simulink model "Modelling"  (R2020a)
settings: Solver=ode4  StartTime=0.0  StopTime=30  FixedStep=0.001  RelTol=1e-3
PreLoadFcn:
  | ControllerToProject.m
values from neighbouring files (symbols this model uses):
  b = 1    [ControllerToProject.m]    (also in Parameters.m)
  g = 9.81    [ControllerToProject.m]    (also in Parameters.m = 9.82)
  l = 0.36022    [ControllerToProject.m]    (also in Parameters.m = 0.35)
  mc = 0.9+0.1    (= 1)    [ControllerToProject.m]    (also in Parameters.m = 0.9)
  mp = 0.08887    [ControllerToProject.m]    (also in Parameters.m = 0.1)
undefined symbols (not defined in the file or in its folder): sigbuilder_block
libraries: simulink x2
settings Model: Creator=Emil  LastModifiedBy=Emil
settings DebuggingCC: ArithmeticOperatorsInVariantConditions=warning
settings SFSimCC: CustomCodeUndefinedFunction=UseInterfaceOnly

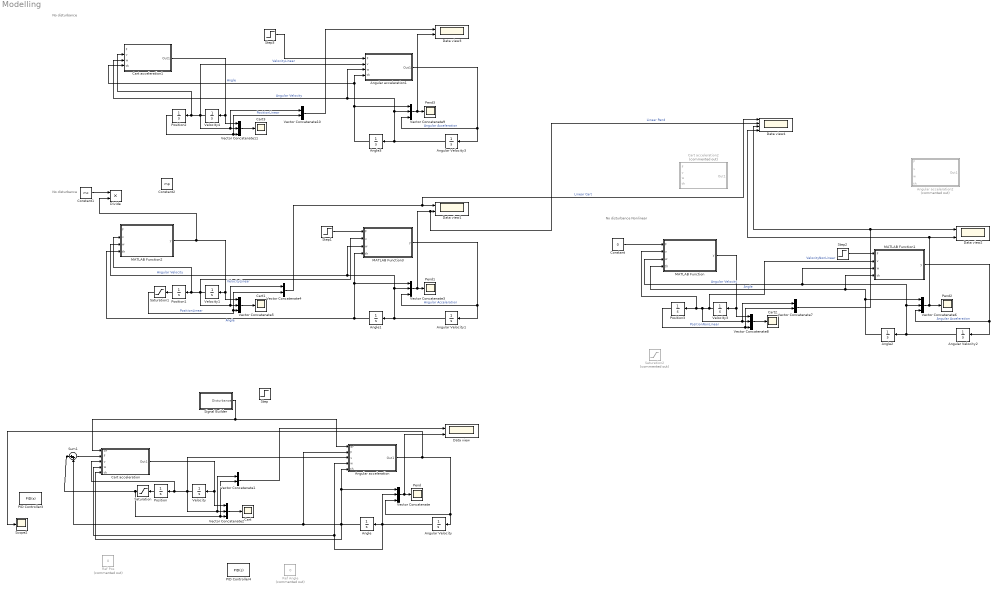
== system Modelling ==
  note: No disturbance
  note: No disturbance
      | Nonlinear
  note: No disturbance
  Angle{,1..3} (4 alike) : Integrator
  Angular Velocity{,1..3} (4 alike) : Integrator
  Angular acceleration : Subsystem
  Angular acceleration1 : Subsystem
  Angular acceleration2 : Subsystem  Commented=on
  Cart{,1..3} (4 alike) : Scope
  Cart acceleration : Subsystem
  Cart acceleration1 : Subsystem
  Cart acceleration2 : Subsystem  Commented=on
  Constant : Constant  Value=0
  Constant1 : Constant  Value=mc
  Constant2 : Constant  Value=mp
  Data view{,1..3} (4 alike) : Scope  NumInputPorts=2
  Data view4 : Scope  NumInputPorts=4
  Divide : Product  Inputs=**
  MATLAB Function : MATLAB Function  TreatAsAtomicUnit=on
  MATLAB Function1 : MATLAB Function  TreatAsAtomicUnit=on
  MATLAB Function2 : MATLAB Function  TreatAsAtomicUnit=on
  MATLAB Function3 : MATLAB Function  TreatAsAtomicUnit=on
  PID Controller3 : simulink/Continuous/PID Controller  Controller=PID  Form=Ideal  TimeDomain=Continuous-time  UseExternalTs=off  SampleTime=-1  IntegratorMethod=Forward Euler  FilterMethod=Forward Euler  ControllerParametersSource=internal  P=-380.892958771882  I=0.42148790930739  D=0.173217560929601  UseFilter=on  N=5979.02668424825  TunerSelectOption=Transfer Function Based (PID Tuner App)  InitialConditionSource=internal  InitialConditionForIntegrator=0  InitialConditionForFilter=0  DifferentiatorICPrevScaledInput=0  ExternalReset=none  TrackingMode=off  Kt=1  LimitOutput=on  UpperSaturationLimit=5  LowerSaturationLimit=-5  LinearizeAsGain=on  AntiWindupMode=clamping  Kb=1  POutMin=[]  POutMax=[]  IOutMin=[]  IOutMax=[]  DOutMin=[]  DOutMax=[]  NOutMin=[]  NOutMax=[]  SumOutMin=[]  SumOutMax=[]  SaturationOutMin=[]  SaturationOutMax=[]  PParamMin=[]  PParamMax=[]  IParamMin=[]  IParamMax=[]  DParamMin=[]  DParamMax=[]  NParamMin=[]  NParamMax=[]  KbParamMin=[]  KbParamMax=[]  KtParamMin=[]  KtParamMax=[]  KbOutMin=[]  KbOutMax=[]  KtOutMin=[]  KtOutMax=[]  IntegratorOutMin=[]  IntegratorOutMax=[]  FilterOutMin=[]  FilterOutMax=[]  SumI1OutMin=[]  SumI1OutMax=[]  SumI2OutMin=[]  SumI2OutMax=[]  SumI3OutMin=[]  SumI3OutMax=[]  SumI4OutMin=[]  SumI4OutMax=[]  SumDOutMin=[]  SumDOutMax=[]  DifferentiatorOutMin=[]  DifferentiatorOutMax=[]  FilterDiffOutCoefMin=[]  FilterDiffOutCoefMax=[]  ReciprocalOutMin=[]  ReciprocalOutMax=[]  SumDenOutMin=[]  SumDenOutMax=[]  SumNumOutMin=[]  SumNumOutMax=[]  DivideOutMin=[]  DivideOutMax=[]  UdiffTsProdOutMin=[]  UdiffTsProdOutMax=[]  NTsProdOutMin=[]  NTsProdOutMax=[]  UintegralTsProdOutMin=[]  UintegralTsProdOutMax=[]  UngainTsProdOutMin=[]  UngainTsProdOutMax=[]  IntegratorContinuousStateAttributes=''  IntegratorStateMustResolveToSignalObject=off  IntegratorRTWStateStorageClass=Auto  FilterContinuousStateAttributes=''  FilterStateMustResolveToSignalObject=off  FilterRTWStateStorageClass=Auto  ParallelPVariant=Passthrough  IdealPVariant=InternalParameters  IVariant=InternalParameters  DVariant=InternalParameters  IntegratorVariant=Continuous  SatVariant=Enabled  AWVariant=ContClampingIdeal  PCopyVariant=InternalParamsIdeal  TRVariant=Disabled  FdbkBlocksVariant=Forward  IdealPFdbkVariant=Disabled  SatFdbkVariant=Disabled  DerivativeFilterVariant=ContFilter  NVariant=InternalParameters  NCopyVariant=Disabled  FilterICVariant=InternalICsFilter  IntegratorICVariant=InternalICs  ExternalResetVariant=Disabled  TRSumVariant=Passthrough  SumFdbkVariant=Disabled  SumVariant=Sum_PID  TsampFilterVariant=InternalTs  TsampNgainVariant=Passthrough  TsampIntegralVariant=Passthrough
  PID Controller4 : simulink/Continuous/PID Controller  Controller=PID  Form=Ideal  TimeDomain=Continuous-time  UseExternalTs=off  SampleTime=-1  IntegratorMethod=Forward Euler  FilterMethod=Forward Euler  ControllerParametersSource=internal  P=-1.40813056601747  I=7297.16708467672  D=0  UseFilter=on  N=100  TunerSelectOption=Transfer Function Based (PID Tuner App)  InitialConditionSource=internal  InitialConditionForIntegrator=0  InitialConditionForFilter=0  DifferentiatorICPrevScaledInput=0  ExternalReset=none  TrackingMode=off  Kt=1  LimitOutput=on  UpperSaturationLimit=5  LowerSaturationLimit=-5  LinearizeAsGain=on  AntiWindupMode=clamping  Kb=1  POutMin=[]  POutMax=[]  IOutMin=[]  IOutMax=[]  DOutMin=[]  DOutMax=[]  NOutMin=[]  NOutMax=[]  SumOutMin=[]  SumOutMax=[]  SaturationOutMin=[]  SaturationOutMax=[]  PParamMin=[]  PParamMax=[]  IParamMin=[]  IParamMax=[]  DParamMin=[]  DParamMax=[]  NParamMin=[]  NParamMax=[]  KbParamMin=[]  KbParamMax=[]  KtParamMin=[]  KtParamMax=[]  KbOutMin=[]  KbOutMax=[]  KtOutMin=[]  KtOutMax=[]  IntegratorOutMin=[]  IntegratorOutMax=[]  FilterOutMin=[]  FilterOutMax=[]  SumI1OutMin=[]  SumI1OutMax=[]  SumI2OutMin=[]  SumI2OutMax=[]  SumI3OutMin=[]  SumI3OutMax=[]  SumI4OutMin=[]  SumI4OutMax=[]  SumDOutMin=[]  SumDOutMax=[]  DifferentiatorOutMin=[]  DifferentiatorOutMax=[]  FilterDiffOutCoefMin=[]  FilterDiffOutCoefMax=[]  ReciprocalOutMin=[]  ReciprocalOutMax=[]  SumDenOutMin=[]  SumDenOutMax=[]  SumNumOutMin=[]  SumNumOutMax=[]  DivideOutMin=[]  DivideOutMax=[]  UdiffTsProdOutMin=[]  UdiffTsProdOutMax=[]  NTsProdOutMin=[]  NTsProdOutMax=[]  UintegralTsProdOutMin=[]  UintegralTsProdOutMax=[]  UngainTsProdOutMin=[]  UngainTsProdOutMax=[]  IntegratorContinuousStateAttributes=''  IntegratorStateMustResolveToSignalObject=off  IntegratorRTWStateStorageClass=Auto  FilterContinuousStateAttributes=''  FilterStateMustResolveToSignalObject=off  FilterRTWStateStorageClass=Auto  ParallelPVariant=Passthrough  IdealPVariant=InternalParameters  IVariant=InternalParameters  DVariant=InternalParameters  IntegratorVariant=Continuous  SatVariant=Enabled  AWVariant=ContClampingIdeal  PCopyVariant=InternalParamsIdeal  TRVariant=Disabled  FdbkBlocksVariant=Forward  IdealPFdbkVariant=Disabled  SatFdbkVariant=Disabled  DerivativeFilterVariant=ContFilter  NVariant=InternalParameters  NCopyVariant=Disabled  FilterICVariant=InternalICsFilter  IntegratorICVariant=InternalICs  ExternalResetVariant=Disabled  TRSumVariant=Passthrough  SumFdbkVariant=Disabled  SumVariant=Sum_PID  TsampFilterVariant=InternalTs  TsampNgainVariant=Passthrough  TsampIntegralVariant=Passthrough
  Pend{,1..3} (4 alike) : Scope
  Position{,1..3} (4 alike) : Integrator
  Ref Angle : Constant  Commented=on  Value=0
  Ref Pos : Constant  Commented=on  Value=0
  Saturation : Saturate  UpperLimit=0.8  LowerLimit=-0.8  LinearizeAsGain=off
  Saturation1 : Saturate  UpperLimit=0.8  LowerLimit=-0.8
  Saturation2 : Saturate  Commented=on  UpperLimit=0.8  LowerLimit=-0.8
  Scope2 : Scope
  Signal Builder : Subsystem  Tag=STV Subsys  LoadFcn=sigbuilder_block('load');  StartFcn=sigbuilder_block('start');  StopFcn=sigbuilder_block('stop');  ClipboardFcn=sigbuilder_block('clipboard');  mask(Sigbuilder block){tuvar=[0:10]}
      mask help: Simulink:masks:SigbuilderBlock_MD
      mask init:
      | if ~strcmp(get_param(bdroot(gcbh),'SimulationStatus'),'stopped') tuvar = sigbuilder_block('maskInit'); end
      settings: CopyFcn=sigbuilder_block('copy');  DeleteFcn=sigbuilder_block('delete');  ModelCloseFcn=sigbuilder_block('modelClose');  PreSaveFcn=sigbuilder_block('preSave');  PauseFcn=sigbuilder_block('pause');  ContinueFcn=sigbuilder_block('continue');  NameChangeFcn=sigbuilder_block('namechange');  OpenFcn=sigbuilder_block('open',[6 30 1428 681.75 ]);  CloseFcn=sigbuilder_block('close');
      mask Display: plot(0, 0, 100, 100,[2, 2, 32, 32, 2], [68, 8, 8, 68, 68],[32, 2], [38, 38], [32, 19, 2],[53, 60, 44], [32, 17, 17, 2],[16, 16, 31, 31]);txt = getActiveGroup(gcbh);text(2, 100, txt,'verticalAlignment', 'top');
  Step : Step  Before=20  After=0  SampleTime=0
  Step1 : Step  Before=20  After=0  SampleTime=0
  Step2 : Step  Before=1  After=0  SampleTime=0
  Step3 : Step  Time=20  Before=1  After=0  SampleTime=0
  Sum1 : Sum  Inputs=|++
  Vector Concatenate{,2..3,5..6,8..9,11} (8 alike) : Concatenate  NumInputs=3
  Vector Concatenate{1,4,7,10} (4 alike) : Concatenate
  Velocity{,1,3..4} (4 alike) : Integrator
  wires:
  Position/1 -> Saturation/1
  Velocity/1 -> Angular acceleration/3(v), Vector Concatenate2/2, Vector Concatenate1/1, Position/1, Cart acceleration/3(v)
  Cart acceleration/1(Out1) -> Velocity/1, Vector Concatenate2/1
  Angular acceleration/1(Out1) -> Scope2/1, Vector Concatenate/3, Angular Velocity/1
  Angular Velocity/1 -> Vector Concatenate/2, Angle/1, Cart acceleration/4(w), Angular acceleration/4(w)
  Saturation/1 -> Sum1/1, Vector Concatenate1/2, Vector Concatenate2/3
  Angle/1 -> Angular acceleration/2(F), Sum1/2, Vector Concatenate/1, Angular acceleration/5(th), Cart acceleration/5(th)
  Vector Concatenate/1 -> Data view/2, Pend/1
  Vector Concatenate2/1 -> Cart/1
  Vector Concatenate1/1 -> Data view/1
  Signal Builder/1(Disturbance) -> Angular acceleration/1(dF), Cart acceleration/1(dF)
  Position1/1 -> Saturation1/1
  Vector Concatenate3/1 -> Data view4/2, Data view1/2, Pend1/1  "Linear Pend"
  Vector Concatenate4/1 -> Data view4/1, Data view1/1  "Linear Cart"
  Vector Concatenate5/1 -> Cart1/1
  Saturation1/1 -> Vector Concatenate4/2, Vector Concatenate5/3  "PositionLinear"
  Angular Velocity1/1 -> Vector Concatenate3/2, MATLAB Function3/3(w), MATLAB Function2/3(w), Angle1/1  "Angular Velocity"
  Velocity1/1 -> MATLAB Function3/2(v), Vector Concatenate4/1, Vector Concatenate5/2, MATLAB Function2/2(v), Position1/1  "VelocityLinear"
  Angle1/1 -> MATLAB Function3/4(th), Vector Concatenate3/1, MATLAB Function2/4(th)  "Angle"
  Angular Velocity2/1 -> MATLAB Function1/3(w), MATLAB Function/3(w), Vector Concatenate6/2, Angle2/1  "Angular Velocity"
  Velocity3/1 -> MATLAB Function1/2(v), Vector Concatenate7/1, Vector Concatenate8/2, MATLAB Function/2(v), Position3/1  "VelocityNonLinear"
  Vector Concatenate6/1 -> Data view2/2, Data view4/4, Pend2/1
  Vector Concatenate8/1 -> Cart2/1
  Vector Concatenate7/1 -> Data view4/3, Data view2/1
  Constant/1 -> MATLAB Function/1(F)
  Position3/1 -> Vector Concatenate7/2, Vector Concatenate8/3  "PositionNonLinear"
  MATLAB Function1/1(y) -> Vector Concatenate6/3, Angular Velocity2/1  "Angular Acceleration"
  MATLAB Function/1(y) -> Vector Concatenate8/1, Velocity3/1
  MATLAB Function2/1(y) -> Divide/2, Velocity1/1, Vector Concatenate5/1
  MATLAB Function3/1(y) -> Vector Concatenate3/3, Angular Velocity1/1  "Angular Acceleration"
  Angle2/1 -> Vector Concatenate6/1, MATLAB Function/4(th), MATLAB Function1/4(th)  "Angle"
  Step2/1 -> MATLAB Function1/1(F)
  Cart acceleration1/1(Out1) -> Velocity4/1, Vector Concatenate11/1
  Vector Concatenate10/1 -> Data view3/1
  Angle3/1 -> Cart acceleration1/4(th), Angular acceleration1/4(th), Vector Concatenate9/1  "Angle"
  Vector Concatenate9/1 -> Data view3/2, Pend3/1
  Step3/1 -> Angular acceleration1/1(F)
  Velocity4/1 -> Angular acceleration1/2(v), Vector Concatenate10/1, Vector Concatenate11/2, Cart acceleration1/2(v), Position2/1  "VelocityLinear"
  Vector Concatenate11/1 -> Cart3/1
  Angular Velocity3/1 -> Vector Concatenate9/2, Cart acceleration1/3(w), Angular acceleration1/3(w), Angle3/1  "Angular Velocity"
  Angular acceleration1/1(Out1) -> Vector Concatenate9/3, Angular Velocity3/1  "Angular Acceleration"
  Position2/1 -> Vector Concatenate10/2, Vector Concatenate11/3  "PositionLinear"
  Sum1/1 -> Cart acceleration/2(F)
  Constant1/1 -> Divide/1
  Step1/1 -> MATLAB Function3/1(F)

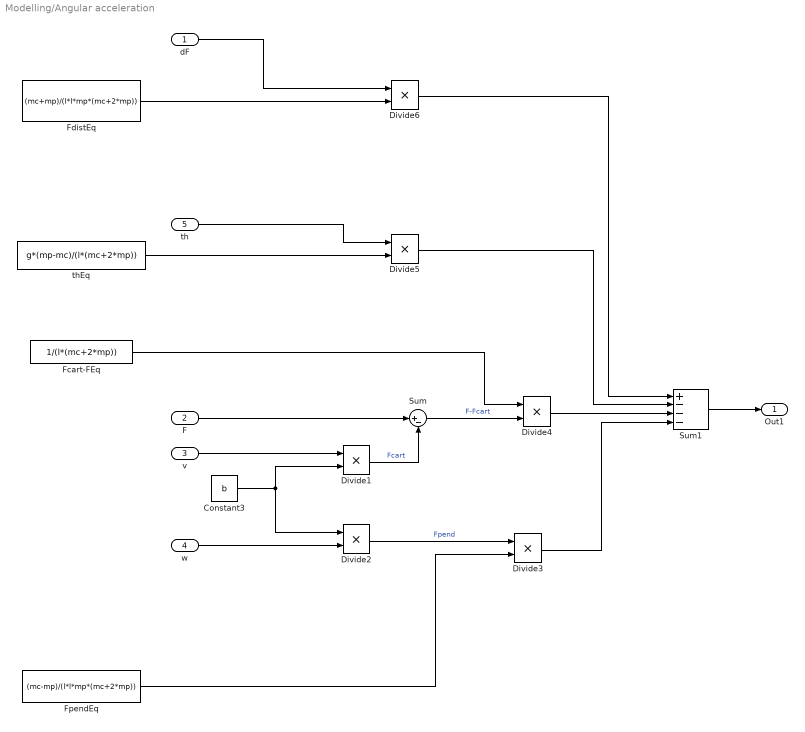
== system Modelling/Angular acceleration ==
  dF : Inport
  F : Inport  Port=2
  v : Inport  Port=3
  w : Inport  Port=4
  th : Inport  Port=5
  Constant3 : Constant  Value=b
  Divide{1..6} (6 alike) : Product  Inputs=**
  Fcart-FEq : Constant  Value=1/(l*(mc+2*mp))
  FdistEq : Constant  Value=(mc+mp)/(l*l*mp*(mc+2*mp))
  FpendEq : Constant  Value=(mc-mp)/(l*l*mp*(mc+2*mp))
  Sum : Sum  Inputs=|+-
  Sum1 : Sum  Inputs=+---
  thEq : Constant  Value=g*(mp-mc)/(l*(mc+2*mp))
  Out1 : Outport
  wires:
  v/1 -> Divide1/1
  Constant3/1 -> Divide2/1, Divide1/2
  w/1 -> Divide2/2
  F/1 -> Sum/1
  Divide1/1 -> Sum/2  "Fcart"
  Divide2/1 -> Divide3/1  "Fpend"
  Sum/1 -> Divide4/2  "F-Fcart"
  th/1 -> Divide5/1
  Divide5/1 -> Sum1/2
  Divide4/1 -> Sum1/3
  Divide3/1 -> Sum1/4
  Sum1/1 -> Out1/1
  dF/1 -> Divide6/1
  Divide6/1 -> Sum1/1
  FpendEq/1 -> Divide3/2
  Fcart-FEq/1 -> Divide4/1
  thEq/1 -> Divide5/2
  FdistEq/1 -> Divide6/2

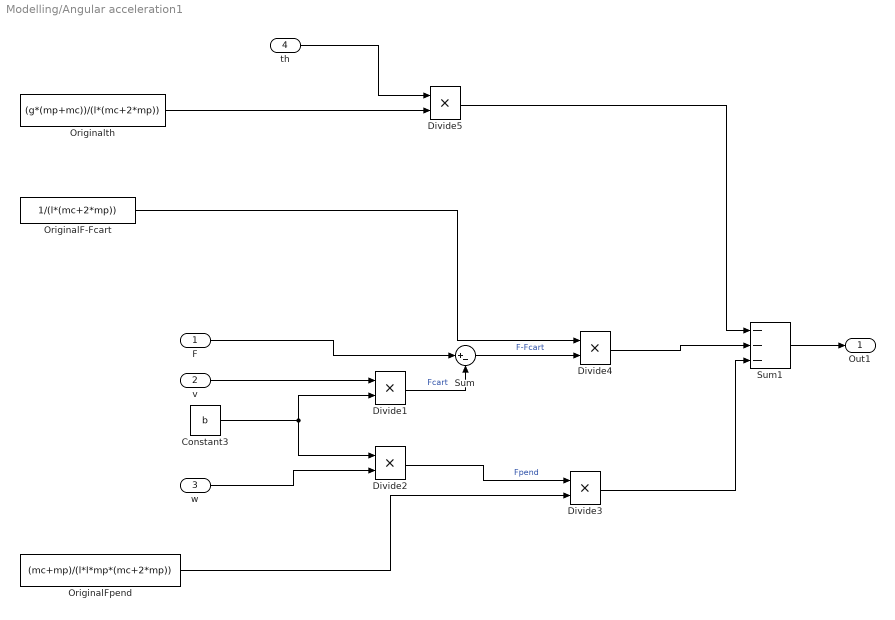
== system Modelling/Angular acceleration1 ==
  F : Inport
  v : Inport  Port=2
  w : Inport  Port=3
  th : Inport  Port=4
  Constant3 : Constant  Value=b
  Divide{1..5} (5 alike) : Product  Inputs=**
  OriginalF-Fcart : Constant  Value=1/(l*(mc+2*mp))
  OriginalFpend : Constant  Value=(mc+mp)/(l*l*mp*(mc+2*mp))
  Originalth : Constant  Value=(g*(mp+mc))/(l*(mc+2*mp))
  Sum : Sum  Inputs=|+-
  Sum1 : Sum  Inputs=---
  Out1 : Outport
  wires:
  v/1 -> Divide1/1
  Constant3/1 -> Divide2/1, Divide1/2
  w/1 -> Divide2/2
  F/1 -> Sum/1
  Divide1/1 -> Sum/2  "Fcart"
  Divide2/1 -> Divide3/1  "Fpend"
  Sum/1 -> Divide4/2  "F-Fcart"
  th/1 -> Divide5/1
  Divide5/1 -> Sum1/1
  Divide4/1 -> Sum1/2
  Divide3/1 -> Sum1/3
  Sum1/1 -> Out1/1
  Originalth/1 -> Divide5/2
  OriginalF-Fcart/1 -> Divide4/1
  OriginalFpend/1 -> Divide3/2

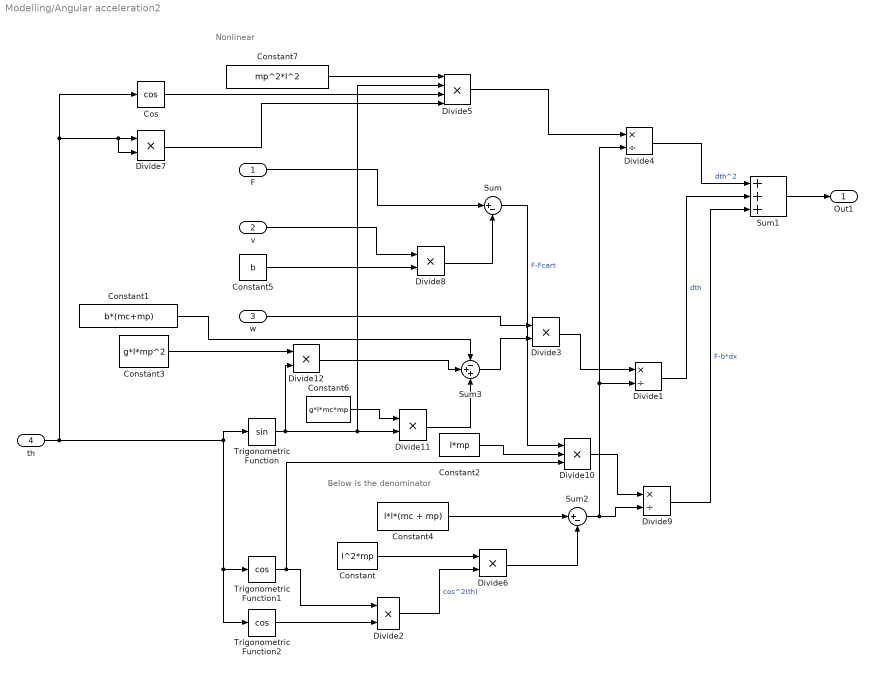
== system Modelling/Angular acceleration2 ==
  note: Below is the denominator
  note: Nonlinear
  F : Inport
  v : Inport  Port=2
  w : Inport  Port=3
  th : Inport  Port=4
  Constant : Constant  Value=l^2*mp
  Constant1 : Constant  Value=b*(mc+mp)
  Constant2 : Constant  Value=l*mp
  Constant3 : Constant  Value=g*l*mp^2
  Constant4 : Constant  Value=l*l*(mc + mp)
  Constant5 : Constant  Value=b
  Constant6 : Constant  Value=g*l*mc*mp
  Constant7 : Constant  Value=mp^2*l^2
  Cos : Trigonometry  Operator=cos
  Divide1 : Product  Inputs=*/
  Divide10 : Product  Inputs=***
  Divide{2..3,6..8,11..12} (7 alike) : Product  Inputs=**
  Divide4 : Product  Inputs=*/
  Divide5 : Product  Inputs=****
  Divide9 : Product  Inputs=*/
  Sum : Sum  Inputs=|+-
  Sum1 : Sum  Inputs=+++
  Sum2 : Sum  Inputs=|+-
  Sum3 : Sum  Inputs=-++
  Trigonometric Function : Trigonometry
  Trigonometric Function1 : Trigonometry  Operator=cos
  Trigonometric Function2 : Trigonometry  Operator=cos
  Out1 : Outport
  wires:
  Divide5/1 -> Divide4/1
  v/1 -> Divide8/1
  Constant5/1 -> Divide8/2
  Sum3/1 -> Divide3/2
  Trigonometric Function/1 -> Divide12/2, Divide11/2, Divide5/2
  Constant/1 -> Divide6/1
  Constant6/1 -> Divide11/1
  Divide2/1 -> Divide6/2  "cos^2(th)"
  Divide10/1 -> Divide9/1
  Divide3/1 -> Divide1/1
  Divide6/1 -> Sum2/2
  Divide8/1 -> Sum/2
  Divide4/1 -> Sum1/1  "dth^2"
  Trigonometric Function2/1 -> Divide2/2
  Sum1/1 -> Out1/1
  Sum/1 -> Divide10/1  "F-Fcart"
  Sum2/1 -> Divide9/2, Divide4/2, Divide1/2
  F/1 -> Sum/1
  w/1 -> Divide3/1
  th/1 -> Divide7/2, Divide7/1, Cos/1, Trigonometric Function1/1, Trigonometric Function2/1, Trigonometric Function/1
  Divide11/1 -> Sum3/3
  Constant7/1 -> Divide5/1
  Constant4/1 -> Sum2/1
  Trigonometric Function1/1 -> Divide10/3, Divide2/1
  Cos/1 -> Divide5/3
  Divide7/1 -> Divide5/4
  Constant2/1 -> Divide10/2
  Divide9/1 -> Sum1/3  "F-b*dx"
  Constant3/1 -> Divide12/1
  Divide12/1 -> Sum3/2
  Constant1/1 -> Sum3/1
  Divide1/1 -> Sum1/2  "dth"

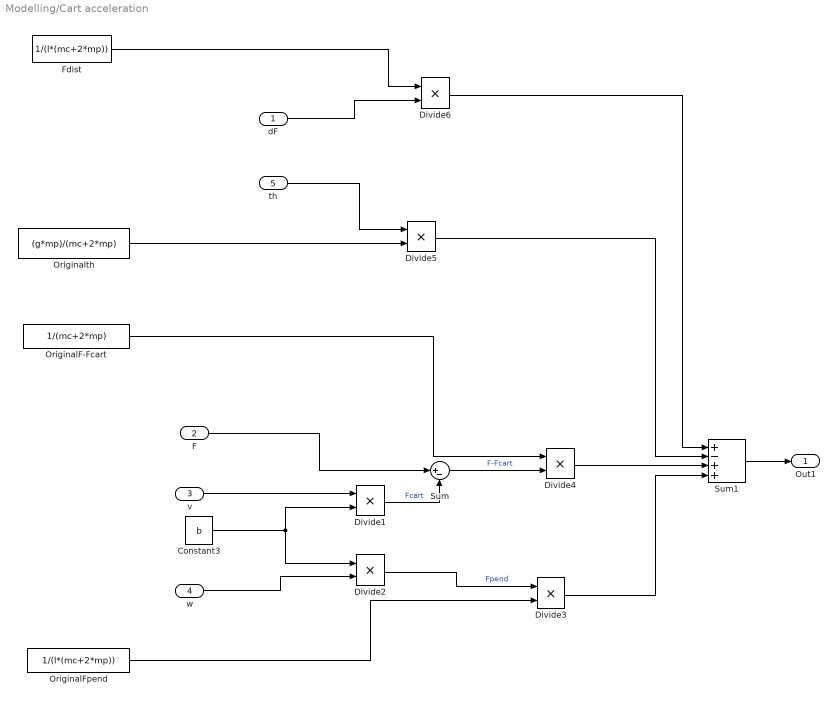
== system Modelling/Cart acceleration ==
  dF : Inport
  F : Inport  Port=2
  v : Inport  Port=3
  w : Inport  Port=4
  th : Inport  Port=5
  Constant3 : Constant  Value=b
  Divide{1..6} (6 alike) : Product  Inputs=**
  Fdist : Constant  Value=1/(l*(mc+2*mp))
  OriginalF-Fcart : Constant  Value=1/(mc+2*mp)
  OriginalFpend : Constant  Value=1/(l*(mc+2*mp))
  Originalth : Constant  Value=(g*mp)/(mc+2*mp)
  Sum : Sum  Inputs=|+-
  Sum1 : Sum  Inputs=+-++
  Out1 : Outport
  wires:
  v/1 -> Divide1/1
  Constant3/1 -> Divide2/1, Divide1/2
  w/1 -> Divide2/2
  F/1 -> Sum/1
  Divide1/1 -> Sum/2  "Fcart"
  Divide2/1 -> Divide3/1  "Fpend"
  Sum/1 -> Divide4/2  "F-Fcart"
  th/1 -> Divide5/1
  Divide5/1 -> Sum1/2
  Divide4/1 -> Sum1/3
  Divide3/1 -> Sum1/4
  Sum1/1 -> Out1/1
  dF/1 -> Divide6/2
  Fdist/1 -> Divide6/1
  OriginalFpend/1 -> Divide3/2
  OriginalF-Fcart/1 -> Divide4/1
  Originalth/1 -> Divide5/2
  Divide6/1 -> Sum1/1

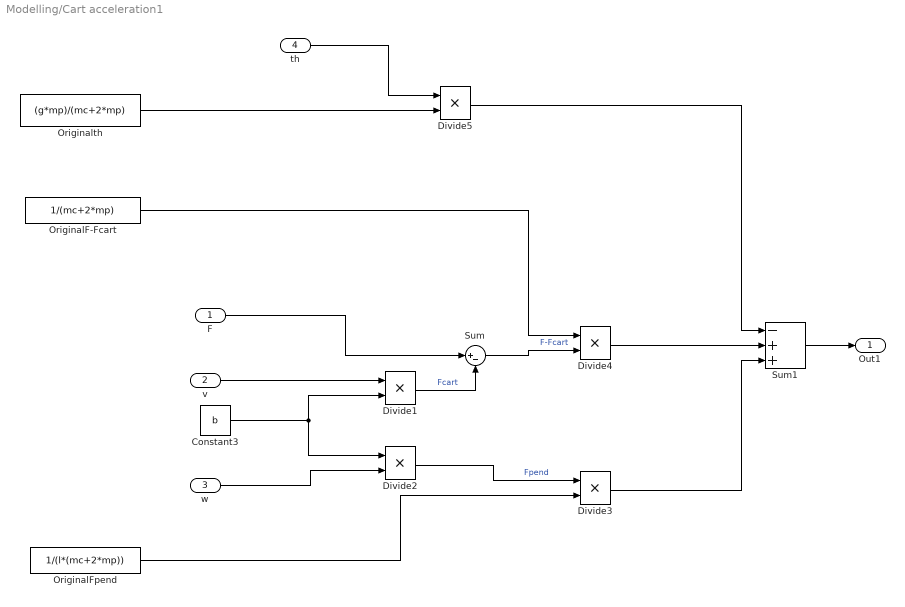
== system Modelling/Cart acceleration1 ==
  F : Inport
  v : Inport  Port=2
  w : Inport  Port=3
  th : Inport  Port=4
  Constant3 : Constant  Value=b
  Divide{1..5} (5 alike) : Product  Inputs=**
  OriginalF-Fcart : Constant  Value=1/(mc+2*mp)
  OriginalFpend : Constant  Value=1/(l*(mc+2*mp))
  Originalth : Constant  Value=(g*mp)/(mc+2*mp)
  Sum : Sum  Inputs=|+-
  Sum1 : Sum  Inputs=-++
  Out1 : Outport
  wires:
  v/1 -> Divide1/1
  Constant3/1 -> Divide2/1, Divide1/2
  w/1 -> Divide2/2
  F/1 -> Sum/1
  Divide1/1 -> Sum/2  "Fcart"
  Divide2/1 -> Divide3/1  "Fpend"
  Sum/1 -> Divide4/2  "F-Fcart"
  th/1 -> Divide5/1
  Divide5/1 -> Sum1/1
  Divide4/1 -> Sum1/2
  Divide3/1 -> Sum1/3
  Sum1/1 -> Out1/1
  OriginalFpend/1 -> Divide3/2
  OriginalF-Fcart/1 -> Divide4/1
  Originalth/1 -> Divide5/2

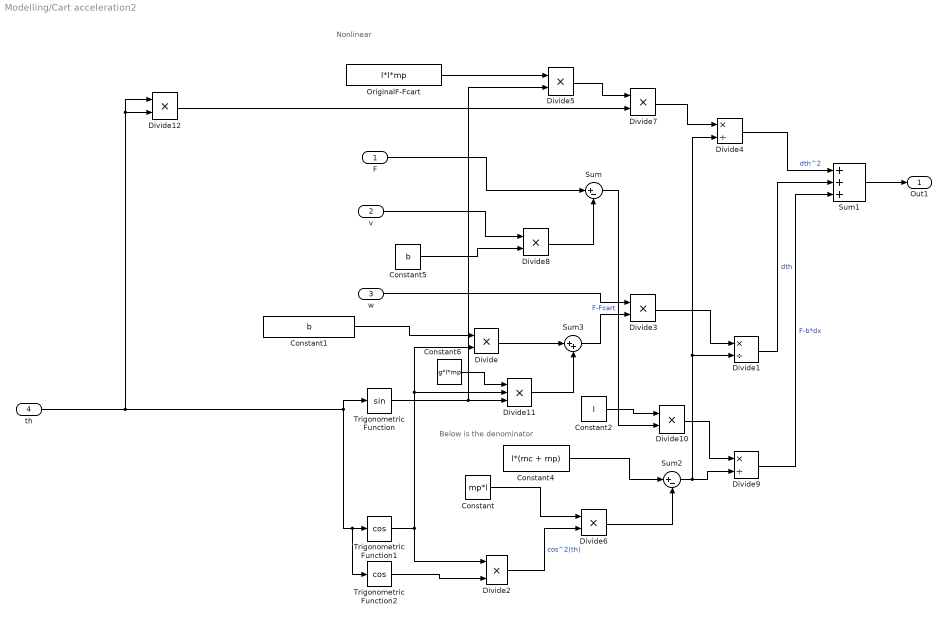
== system Modelling/Cart acceleration2 ==
  note: Below is the denominator
  note: Nonlinear
  F : Inport
  v : Inport  Port=2
  w : Inport  Port=3
  th : Inport  Port=4
  Constant : Constant  Value=mp*l
  Constant1 : Constant  Value=b
  Constant2 : Constant  Value=l
  Constant4 : Constant  Value=l*(mc + mp)
  Constant5 : Constant  Value=b
  Constant6 : Constant  Value=g*l*mp
  Divide{,2..3,5..8,10,12} (9 alike) : Product  Inputs=**
  Divide1 : Product  Inputs=*/
  Divide11 : Product  Inputs=***
  Divide4 : Product  Inputs=*/
  Divide9 : Product  Inputs=*/
  OriginalF-Fcart : Constant  Value=l*l*mp
  Sum : Sum  Inputs=|+-
  Sum1 : Sum  Inputs=+++
  Sum2 : Sum  Inputs=|+-
  Sum3 : Sum  Inputs=|++
  Trigonometric Function : Trigonometry
  Trigonometric Function1 : Trigonometry  Operator=cos
  Trigonometric Function2 : Trigonometry  Operator=cos
  Out1 : Outport
  wires:
  w/1 -> Divide3/1
  F/1 -> Sum/1
  Sum/1 -> Divide10/2  "F-Fcart"
  Sum1/1 -> Out1/1
  th/1 -> Divide12/1, Divide12/2, Trigonometric Function2/1, Trigonometric Function1/1, Trigonometric Function/1
  Constant1/1 -> Divide/1
  Trigonometric Function1/1 -> Divide11/2, Divide/2, Divide2/1
  Trigonometric Function2/1 -> Divide2/2
  Constant/1 -> Divide6/1
  Divide2/1 -> Divide6/2  "cos^2(th)"
  Divide6/1 -> Sum2/2
  Constant4/1 -> Sum2/1
  Constant5/1 -> Divide8/2
  v/1 -> Divide8/1
  Sum2/1 -> Divide9/2, Divide4/2, Divide1/2
  Constant2/1 -> Divide10/1
  Divide8/1 -> Sum/2
  Divide10/1 -> Divide9/1
  Divide9/1 -> Sum1/3  "F-b*dx"
  Constant6/1 -> Divide11/1
  Trigonometric Function/1 -> Divide5/2, Divide11/3
  Divide11/1 -> Sum3/2
  Divide/1 -> Sum3/1
  Sum3/1 -> Divide3/2
  Divide3/1 -> Divide1/1
  Divide1/1 -> Sum1/2  "dth"
  OriginalF-Fcart/1 -> Divide5/1
  Divide4/1 -> Sum1/1  "dth^2"
  Divide5/1 -> Divide7/1
  Divide12/1 -> Divide7/2
  Divide7/1 -> Divide4/1

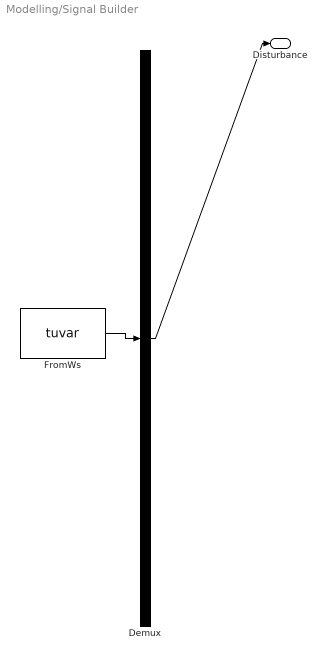
== system Modelling/Signal Builder ==
  Demux : Demux  Tag=STV Demux  Outputs=1
      settings: DisplayOption=none
  FromWs : FromWorkspace  Tag=STV FromWs  VariableName=tuvar
      SigBuilderData=|
      | common.afterFinalStr = 'Extrapolate'
      | common.sampleTime = 0
      | dataSet.timeRange = [0 10]
      | dataSet.name = 'Group 1'
      | sbobj.Groups.Name = 'Group 1'
      | sbobj.Groups.Signals.Name = 'Disturbance'
      | sbobj.Groups.Signals.XData = [0 0.25 0.5 0.75 1 1.25 1.5 1.75 2 2.25 2.5 2.75 3 3.25 3.5 3.75 4 4.25 4.5 4.75 5 5.25 5.5 5.75 6 6.25 6.5 6.75 7 7.25 7.5 7.75 8 8.25 8.5 8.75 9 9.25 9.5 9.75 10]
      | sbobj.Groups.Signals.YData = [0 0 0 0 0 0 0 0 0 0 0 -2.77555756156e-17 -0.002 0.063 0.002 -0.03 -0.05 -0.05 0.01 -0.146 0.16 0.08 0.1 0.089 0.193 0.06 0.02 -2.7756e-18 -0.022 -0.034 -0.099 -0.084 -0.01 -0.02 -0.051 -0.045 0.02 0.02 0.176 -2.7756e-18 -2.77555756156e-17]
  Disturbance : Outport  Tag=STV Outport
  wires:
  FromWs/1 -> Demux/1
  Demux/1 -> Disturbance/1

== matlab function Modelling/MATLAB Function1 ==
  data: F input; y output; v input; w input; th input
function y = ddthPendNonLin(F, v, w, th)
mc=0.9+0.1; 
mp=0.08887;
l= 0.36022;
g = 9.81;
b = 8.2;

y = -(b*w*mc + b*w*mp + F*l*mp*cos(th) - g*l*mp^2*sin(th) + w^2*l^2*mp^2*cos(th)*sin(th) - b*v*l*mp*cos(th) - g*l*mc*mp*sin(th))/(l^2*mp*(- mp*cos(th)^2 + mc + mp));

== matlab function Modelling/MATLAB Function ==
  data: F input; y output; v input; w input; th input
function y = ddxCartnonLin(F, v, w, th)

mc=0.9+0.1; 
mp=0.08887;
l= 0.36022;
g = 9.81;
b = 8.2;

y = (F*l - b*v*l + b*w*cos(th) + w^2*l^2*mp*sin(th) - g*l*mp*cos(th)*sin(th))/(l*(- mp*cos(th)^2 + mc + mp));

== matlab function Modelling/MATLAB Function2 ==
  data: F input; y output; v input; w input; th input
function y = ddxCartLin(F, v, w, th)

mc=0.9+0.1; 
mp=0.08887;
l= 0.36022;
g = 9.81;
b = 8.2;

y = ((b*w) + F*l - (b*v)*l - g*l*mp*th)/(l*(mc + 2*mp));

== matlab function Modelling/MATLAB Function3 ==
  data: F input; y output; v input; w input; th input
function y = ddthPend(F, v, w, th)
mc=0.9+0.1; 
mp=0.08887;
l= 0.36022;
g = 9.81;
b = 8.2;

y = -((b*w)*mc + (b*w)*mp - F*l*mp + (b*v)*l*mp - g*l*mp^2*th - g*l*mc*mp*th)/(l^2*mp*(mc + 2*mp));
